simulink model "DSSSusingBPSK"  (R2020a)
settings: Solver=FixedStepAuto  StartTime=0.0  StopTime=10.0  FixedStep=0.01  RelTol=1e-3
libraries: commseqgen3 x1
settings Model: Creator=AVS  LastModifiedBy=AVS

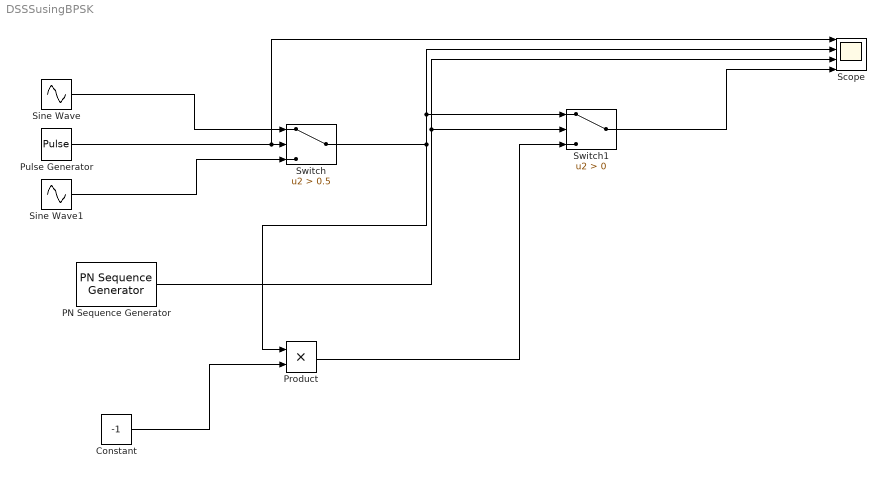
== system DSSSusingBPSK ==
  Constant : Constant  Value=-1
  PN Sequence Generator : commseqgen3/PN Sequence Generator  poly='z^6 + z + 1'  ini_sta=[0 0 0 0 0 1]  outBitMaskSource=Dialog parameter  shift=0  outVarSiz=off  maxOutSizeMode=Dialog parameter  maxOutSize=[10 1]  Ts=1  sampPerFrame=1  reset=off  bitPackedOutputs=off  outDataType=double  numPackedBits=8  bitPackDataSigned=off  bitPackedOutDType=double
  Product : Product
  Pulse Generator : DiscretePulseGenerator  PulseType=Time based  PulseWidth=50
  Scope : Scope  NumInputPorts=4
  Sine Wave : Sin  Frequency=2*pi*4  SampleTime=0.01
  Sine Wave1 : Sin  Frequency=2*pi*4  Phase=pi  SampleTime=0.01
  Switch : Switch  Criteria=u2 > Threshold  Threshold=0.5
  Switch1 : Switch  Criteria=u2 > Threshold
  wires:
  Pulse Generator/1 -> Scope/1, Switch/2
  Sine Wave1/1 -> Switch/3
  Sine Wave/1 -> Switch/1
  Switch/1 -> Product/1, Scope/2, Switch1/1
  PN Sequence Generator/1 -> Scope/3, Switch1/2
  Constant/1 -> Product/2
  Product/1 -> Switch1/3
  Switch1/1 -> Scope/4
